simulink subsystem "Compression"  (R2024b)
settings: Solver=VariableStepAuto  StartTime=0.0  StopTime=10.0  RelTol=1e-3
settings Model: Creator=The MathWorks, Inc.  LastModifiedBy=The MathWorks, Inc.

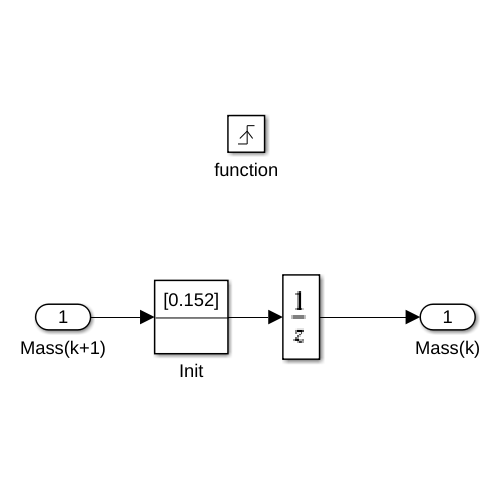
[thumbnail: Simulink's stored preview of the top-level diagram]
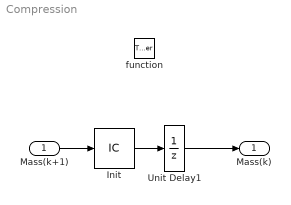
== system Compression ==
  Mass(k+1) : Inport
  function : TriggerPort  VariantControl=(inherit)  InitialTriggerSignalState=zero
  Init : InitialCondition  Value=0.152
  Unit Delay1 : UnitDelay  InitialCondition=0.152  SampleTime=-1  HasFrameUpgradeWarning=on
  Mass(k) : Outport  InitialOutput=0.152  VectorParamsAs1DForOutWhenUnconnected=off
  wires:
  Unit Delay1/1 -> Mass(k)/1
  Init/1 -> Unit Delay1/1
  Mass(k+1)/1 -> Init/1
